simulink model "mag_mtq_duty_cycle_mag_hold_test"  (R2018b)
settings: Solver=FixedStepAuto  StartTime=0.0  StopTime=10.0  FixedStep=fswParams.sample_time_s  RelTol=1e-3
libraries: mag_mtq_duty_cycle_lib x1
settings Model: Creator=Taylor  LastModifiedBy=Taylor

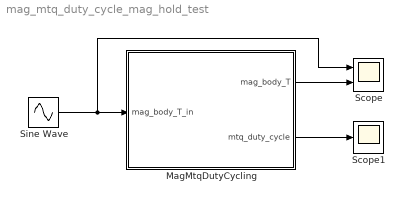
== system mag_mtq_duty_cycle_mag_hold_test ==
  MagMtqDutyCycling : Subsystem  AncestorBlock=MEKF_Conversion_lib/Conversion_lib/MagMtqDutyCycling
  Scope : Scope  NumInputPorts=2
  Scope1 : Scope
  Sine Wave : Sin  SampleTime=0
  wires:
  Sine Wave/1 -> Scope/1, MagMtqDutyCycling/1(mag_body_T_in)
  MagMtqDutyCycling/2(mtq_duty_cycle) -> Scope1/1
  MagMtqDutyCycling/1(mag_body_T) -> Scope/2

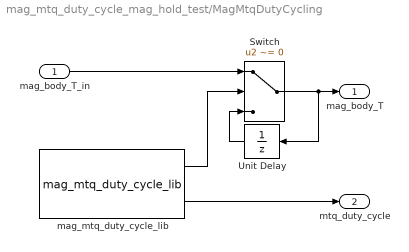
== system mag_mtq_duty_cycle_mag_hold_test/MagMtqDutyCycling ==
  mag_body_T_in : Inport
  Switch : Switch  Criteria=u2 ~= 0  OutDataTypeStr=double  InputSameDT=on
  Unit Delay : UnitDelay  SampleTime=-1
  mag_mtq_duty_cycle_lib : mag_mtq_duty_cycle_lib/mag_mtq_duty_cycle_lib  SystemSampleTime=-1
  mag_body_T : Outport
  mtq_duty_cycle : Outport  Port=2
  wires:
  mag_mtq_duty_cycle_lib/1 -> Switch/2
  mag_mtq_duty_cycle_lib/2 -> mtq_duty_cycle/1
  mag_body_T_in/1 -> Switch/1
  Unit Delay/1 -> Switch/3
  Switch/1 -> Unit Delay/1, mag_body_T/1
